simulink model "test_RehaMove3"  (R2016b)
settings: Solver=FixedStepDiscrete  StartTime=0.0  StopTime=inf  FixedStep=0.04  RelTol=1e-3
libraries: simulink x2, LIB_RehaMovePro x1
settings Model: SimulationMode=external  ExtModeTrigDuration=10000  Creator=constantin  LastModifiedBy=valtin
settings DataIOCC: LimitDataPoints=on  SaveFormat=Array
settings OptimizationCC: ExpressionDepthLimit=2147483647  LifeSpan=1
settings DebuggingCC: UnderspecifiedInitializationDetection=Classic  MergeDetectMultiDrivingBlocksExec=none  SolverPrmCheckMsg=warning  StateNameClashWarn=warning  SFUnexpectedBacktrackingDiag=warning  SFNoUnconditionalDefaultTransitionDiag=warning  SFExecutionAtInitializationDiag=none
settings HardwareCC: ProdBitPerPointer=32  ProdBitPerSizeT=32  ProdBitPerPtrDiffT=32  ProdLargestAtomicFloat=None  ProdIntDivRoundTo=Undefined  ProdEndianess=Unspecified  ProdWordSize=32  ProdHWDeviceType=32-bit Generic
settings ModelReferenceCC: PropagateSignalLabelsOutOfModel=off
settings SFSimCC: SimCustomHeaderCode="#include \"rehamove.hpp\""
settings SFSimCC: SimUserIncludeDirs=|
  | /Users/constantin/Documents/retrainer/retrainer.repo/code/trunk/incl/rehamove/
  | /Users/constantin/Documents/retrainer/retrainer.repo/code/trunk/incl/
settings RTWCC: SystemTargetFile=ert_linux.tlc  MakeCommand=make_rtw OPTS=-DWITH_HW OPTIMIZATION_FLAGS=-O3  TemplateMakefile=ert_linux.tmf  Description=Linux Embedded Coder  TargetLang=C++
settings CodeAppCC: IgnoreCustomStorageClasses=off  CustomSymbolStrType=$N$R$M  InternalIdentifier=Classic
settings STFCustomTargetCC: ModelReferenceCompliant=off  GeneratePreprocessorConditionals=Disable all  CombineOutputUpdateFcns=on  ERTCustomFileBanners=on  SupportComplex=off  RemoveResetFunc=on  SupportVariableSizeSignals=on  MATLABClassNameForMDSCustomization=Simulink.SoftwareTarget.ERTCustomization  GRTInterface=off  SystemTargetFile=ert_linux.tlc
settings ERTTargetCC: ModelReferenceCompliant=off  ParMdlRefBuildCompliant=off  CompOptLevelCompliant=off  ConcurrentExecutionCompliant=off  GeneratePreprocessorConditionals=Disable all  ERTFirstTimeCompliant=off  SupportComplex=off  SupportContinuousTime=on  SupportNonInlinedSFcns=on  SupportVariableSizeSignals=on  ModelStepFunctionPrototypeControlCompliant=off  CPPClassGenCompliant=off  UseToolchainInfoCompliant=off  ExtMode=on  MultiInstanceErrorCode=None  ERTCustomFileTemplate=ert_linux_file_process.tlc  ConvertIfToSwitch=off  SuppressUnreachableDefaultCases=off
settings ConfigComp: CovMetricSettings=dw  CovHtmlReporting=on  CovSaveCumulativeToWorkspaceVar=on  CovSaveSingleToWorkspaceVar=on  CovExternalEMLEnable=off  CovSFcnEnable=off
settings ConfigurationSet: Description=SimMechanics 2G

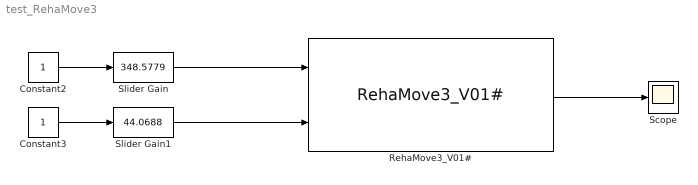
== system test_RehaMove3 ==
  Constant2 : Constant  OutDataTypeStr=double  SampleTime=0.04
  Constant3 : Constant  OutDataTypeStr=double  SampleTime=0.04
  RehaMove3_V01# : LIB_RehaMovePro/RehaMove3_V01#  stimDevicePath=/dev/ttyUSB0  stimDeviceSerial=170150003  stimChannels="[ 2  ]"  stimFrequency=25  stimRehaMoveProProtocol="Use the LowLevel protocol   -> Each stimulation pulse is send separatly."  stimMaxCurrent=120  stimMaxPulsWidth=500  stimBlockID=STIM1  stimTextSampleTime=0.04s (based on stimulation frequency)  SampleTime=0.04  stimThreadInit=on  stimThreadData=on  stimAbortError=3  stimTestAgain=2  llPulseShape=[15]  llNumberOfParts=1  llMaxStimVoltage=90V  llActivateDenervation=off  Parameter58=0  miscPrintBlockParam=off  miscPrintDeviceInfos=off  miscPrintSendInfos=off  miscPrintReceiveInfos=off  miscPrintInitInfos=off  miscPrintStimInfos=on  miscPrintRMPInitSettings=on  miscPrintSequenceErrors=on  miscPrintCorrectionChargeWarnings=on  miscPrintStats=on  miscUseColors=on  miscEnableAdvancedSettings=on  miscDisableVersionCheck=off
  Scope : Scope
  Slider Gain : simulink/Math Operations/Slider Gain  low=0  gain=348.5779  high=510
  Slider Gain1 : simulink/Math Operations/Slider Gain  low=0  gain=44.0688  high=130
  wires:
  RehaMove3_V01#/1 -> Scope/1
  Slider Gain/1 -> RehaMove3_V01#/1
  Slider Gain1/1 -> RehaMove3_V01#/2
  Constant2/1 -> Slider Gain/1
  Constant3/1 -> Slider Gain1/1
